simulink model "test_Addiction"  (R2018b)
settings: Solver=FixedStepDiscrete  StartTime=0.0  StopTime=10.0  RelTol=1e-3
libraries: autosarspkglib x2
settings Model: Creator=ganya  LastModifiedBy=ganya
settings OptimizationCC: DefaultParameterBehavior=Inlined  EnhancedBackFolding=on  PassReuseOutputArgsAs=Individual arguments  ZeroExternalMemoryAtStartup=off  ZeroInternalMemoryAtStartup=off  OptimizeBlockOrder=speed  DifferentSizesBufferReuse=on  OptimizationCustomize=off
settings DebuggingCC: ParameterTunabilityLossMsg=error
settings SFSimCC: MATLABDynamicMemAlloc=off
settings RTWCC: SystemTargetFile=autosar.tlc  GenCodeOnly=on  TemplateMakefile=ert_default_tmf  Description=AUTOSAR  GenerateReport=on  IncludeHyperlinkInReport=on  LaunchReport=on  GenerateTraceInfo=on  GenerateTraceReport=on  GenerateTraceReportSl=on  GenerateTraceReportSf=on  GenerateTraceReportEml=on
settings CodeAppCC: ForceParamTrailComments=on  IgnoreCustomStorageClasses=off  OperatorAnnotations=on  SimulinkDataObjDesc=on  SFDataObjDesc=on  InsertBlockDesc=on
settings STFCustomTargetCC: TargetLangStandard=C99 (ISO)  MultiwordLength=256  ParMdlRefBuildCompliant=on  CompOptLevelCompliant=on  CombineOutputUpdateFcns=on  SuppressErrorStatus=on  ERTCustomFileBanners=on  SupportNonFinite=off  SupportComplex=off  SupportContinuousTime=off  SupportNonInlinedSFcns=off  RemoveResetFunc=on  MATLABClassNameForMDSCustomization=Simulink.SoftwareTarget.ERTCustomization  AutosarCompliant=on  UseToolchainInfoCompliant=on  LookupTableObjectStructAxisOrder=2,1,3,4,...  LUTObjectStructOrderEvenSpacing=Size,Table,Breakpoints  SystemTargetFile=autosar.tlc
settings ERTTargetCC: TargetLangStandard=C99 (ISO)  ConcurrentExecutionCompliant=off  SuppressErrorStatus=on  SupportNonFinite=off  SupportComplex=off  ModelStepFunctionPrototypeControlCompliant=off  CPPClassGenCompliant=off  AutosarCompliant=on  LookupTableObjectStructAxisOrder=2,1,3,4,...  LUTObjectStructOrderEvenSpacing=Size,Table,Breakpoints  InlinedParameterPlacement=NonHierarchical  ERTCustomFileTemplate=example_file_process.tlc

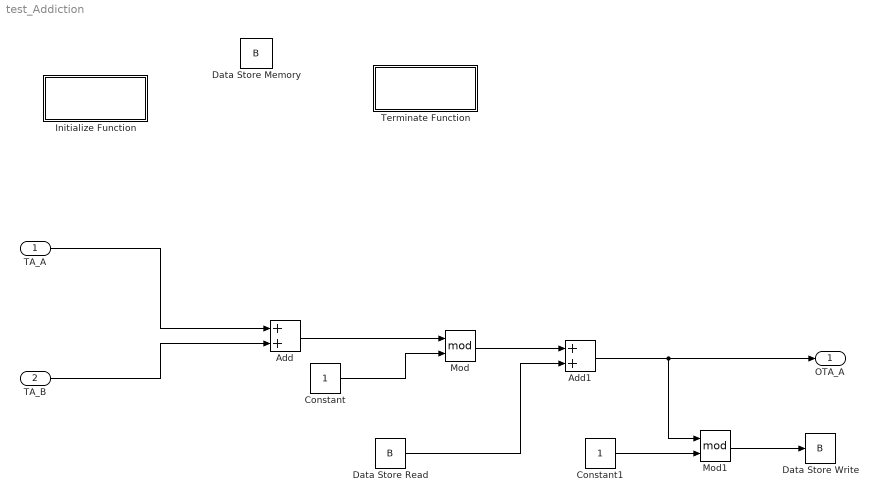
== system test_Addiction ==
  TA_A : Inport
  TA_B : Inport  Port=2
  Add : Sum
  Add1 : Sum
  Constant : Constant  OutDataTypeStr=uint8
  Constant1 : Constant  OutDataTypeStr=uint8
  Data Store Memory : DataStoreMemory  DataStoreName=B  ReadBeforeWriteMsg=warning  WriteAfterWriteMsg=warning  WriteAfterReadMsg=warning  ShowAdditionalParam=off
  Data Store Read : DataStoreRead  DataStoreName=B
  Data Store Write : DataStoreWrite  DataStoreName=B
  Initialize Function : Subsystem  TreatAsAtomicUnit=on
  Mod : Math  Operator=mod  SaturateOnIntegerOverflow=on
  Mod1 : Math  Operator=mod  SaturateOnIntegerOverflow=on
  Terminate Function : Subsystem  TreatAsAtomicUnit=on
  OTA_A : Outport
  wires:
  TA_A/1 -> Add/1
  TA_B/1 -> Add/2
  Add/1 -> Mod/1
  Constant/1 -> Mod/2
  Mod/1 -> Add1/1
  Data Store Read/1 -> Add1/2
  Add1/1 -> Mod1/1, OTA_A/1
  Constant1/1 -> Mod1/2
  Mod1/1 -> Data Store Write/1

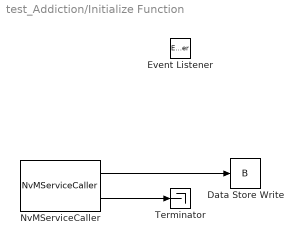
== system test_Addiction/Initialize Function ==
  Data Store Write : DataStoreWrite  DataStoreName=B
  Event Listener : EventListener  DisableCoverage=on  EventName=reset
  NvMServiceCaller : autosarspkglib/Basic Software/NVRAM Manager (NvM)/NvMServiceCaller  PortName=Eep_B  Operation=ReadBlock  ArgumentSpecification=uint8(1)  st=-1  ServiceImpl=autosar.bsw.NvMService
      settings: SourceProductName=Embedded Coder Support Package for AUTOSAR Standard  SourceProductBaseCode=EC_AUTOSAR
  Terminator : Terminator
  wires:
  NvMServiceCaller/1 -> Data Store Write/1
  NvMServiceCaller/2 -> Terminator/1

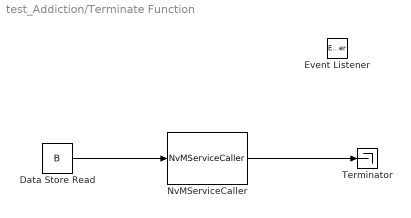
== system test_Addiction/Terminate Function ==
  Data Store Read : DataStoreRead  DataStoreName=B
  Event Listener : EventListener  DisableCoverage=on  EventType=Terminate  EventName=reset
  NvMServiceCaller : autosarspkglib/Basic Software/NVRAM Manager (NvM)/NvMServiceCaller  PortName=NvMService  Operation=WriteBlock  ArgumentSpecification=uint8(1)  st=-1  ServiceImpl=autosar.bsw.NvMService
      settings: SourceProductName=Embedded Coder Support Package for AUTOSAR Standard  SourceProductBaseCode=EC_AUTOSAR
  Terminator : Terminator
  wires:
  Data Store Read/1 -> NvMServiceCaller/1
  NvMServiceCaller/1 -> Terminator/1
